simulink model "Simulink_1"  (R2018a)
settings: Solver=VariableStepAuto  StartTime=0.0  StopTime=50  RelTol=1e-3
libraries: dspsrcs4 x1
settings Model: Creator=student  LastModifiedBy=student

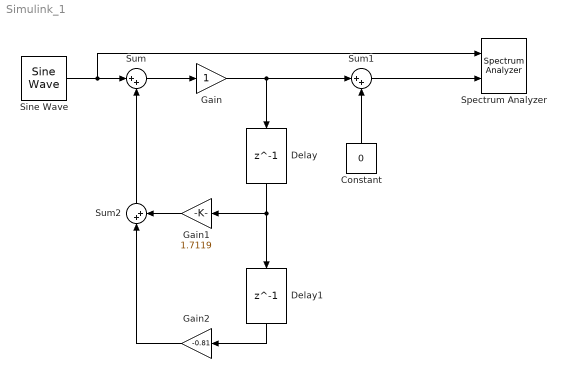
== system Simulink_1 ==
  Constant : Constant  Value=0  SampleTime=1
  Delay : Delay  DelayLength=1
  Delay1 : Delay  DelayLength=1
  Gain : Gain  RndMeth=Zero  ParamDataTypeStr=Inherit: Same as input
  Gain1 : Gain  Gain=1.7119  RndMeth=Zero  ParamDataTypeStr=Inherit: Same as input
  Gain2 : Gain  Gain=-0.81  RndMeth=Zero  OutDataTypeStr=Inherit: Same as input  ParamDataTypeStr=Inherit: Same as input
  Sine Wave : dspsrcs4/Sine Wave  Amplitude=1  Frequency=5  Phase=0  SampleMode=Discrete  OutComplex=Real  CompMethod=Table lookup  TableSize=Speed  SampleTime=1/100  SamplesPerFrame=1  ResetState=Restart at time zero  OutputFrames=off  dataType=double  wordLen=16  udDataType=sfix(16)  fracBitsMode=Best precision  numFracBits=15  OutDataTypeStr=double  LastOutDataTypeStr=double
  Spectrum Analyzer : SpectrumAnalyzer  NumInputPorts=2
  Sum : Sum  Inputs=|++
  Sum1 : Sum  Inputs=|++
  Sum2 : Sum  Inputs=|++
  wires:
  Sine Wave/1 -> Spectrum Analyzer/1, Sum/1
  Sum/1 -> Gain/1
  Gain/1 -> Delay/1, Sum1/1
  Constant/1 -> Sum1/2
  Sum2/1 -> Sum/2
  Delay/1 -> Delay1/1, Gain1/1
  Gain1/1 -> Sum2/2
  Delay1/1 -> Gain2/1
  Gain2/1 -> Sum2/1
  Sum1/1 -> Spectrum Analyzer/2
